simulink model "inv_rot_pen_RL_cntr_simscape_sim_1d_analysis"  (R2025b)
settings: Solver=FixedStepAuto  StartTime=0.0  StopTime=5  FixedStep=Ts  RelTol=1e-3
StopFcn:
  | myStopFcnAppendInitTime
values from neighbouring files (symbols this model uses):
  cfg = loaded.cfg    [continueFurutaMatlabSwingupTraining.m]    (also in evaluateFurutaController.m = makeFurutaConfig(); evaluateFurutaMatlabSwingupAgent.m = makeFurutaMatlabSwingupTD3Config(); finalizeFurutaDirectTD3Run.m = normalizeRunConfig(cfg, runDir); initFurutaSldrtHardwareWorkspace.m = makeFurutaMathWorksStyleWideTD3Config())
  i_max = 4    [initFurutaModelWorkspace.m]
  K = K_oben    [initFurutaModelWorkspace.m]
  Kp_i = db2mag(options.CurrentControllerKpDb)    [initFurutaModelWorkspace.m]    (also in initFurutaSldrtHardwareWorkspace.m = 2.5)
  omega0 = options.InitialOmega    [initFurutaModelWorkspace.m]
  param = get_parameter()    [initFurutaModelWorkspace.m]
  s = zpk("s")    [initFurutaModelWorkspace.m]    (also in initFurutaSldrtHardwareWorkspace.m)
  theta0 = options.InitialTheta    [initFurutaModelWorkspace.m]
  Tn_i = param.L / param.R    [initFurutaModelWorkspace.m]    (also in initFurutaSldrtHardwareWorkspace.m = 0.000286849073257)
  Ts_fast = cfg.Model.HardwareFastSampleTime    [initFurutaSldrtHardwareWorkspace.m]
undefined symbols (not defined in the file or in its folder): currentBias_A, currentNoiseStd_A, DiscIntNeverNeededParam, G_diff_theta1_ss, G_diff_theta2, G_diff_theta2_ss, G_encoder_notch_d_ss, rewardParams, safetyParams, X, Y, Z
libraries: sm_lib x57, nesl_utility x18, cstblocks x13, rllib x2, simulink x1
(part 3 of 3)

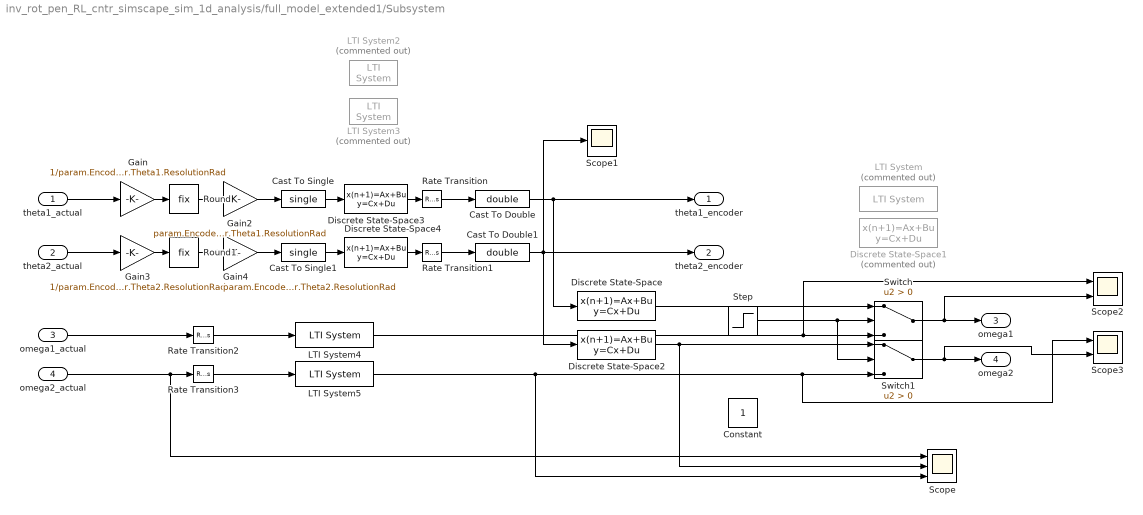
== system inv_rot_pen_RL_cntr_simscape_sim_1d_analysis/full_model_extended1/Subsystem ==
  theta1_actual : Inport
  theta2_actual : Inport  Port=2
  omega1_actual : Inport  Port=3
  omega2_actual : Inport  Port=4
  Cast To Double : DataTypeConversion  OutDataTypeStr=double  SaturateOnIntegerOverflow=off  RndMeth=Floor
  Cast To Double1 : DataTypeConversion  OutDataTypeStr=double  SaturateOnIntegerOverflow=off  RndMeth=Floor
  Cast To Single : DataTypeConversion  OutDataTypeStr=single  SaturateOnIntegerOverflow=off  RndMeth=Floor
  Cast To Single1 : DataTypeConversion  OutDataTypeStr=single  SaturateOnIntegerOverflow=off  RndMeth=Floor
  Constant : Constant
  Discrete State-Space : DiscreteStateSpace  A=G_diff_theta1_ss.A  B=G_diff_theta1_ss.B  C=G_diff_theta1_ss.C  D=G_diff_theta1_ss.D  InitialCondition=|  SampleTime=cfg.Agent.SampleTime
      | rampConsistentFilterX0( ...
      |     G_diff_theta1_ss, theta0(1), omega0(1), cfg.Agent.SampleTime);
  Discrete State-Space1 : DiscreteStateSpace  Commented=on  A=G_diff_theta2.A  B=G_diff_theta2.B  C=G_diff_theta2.C  D=G_diff_theta2.D  InitialCondition=2.78824  SampleTime=cfg.Agent.SampleTime
  Discrete State-Space2 : DiscreteStateSpace  A=G_diff_theta2_ss.A  B=G_diff_theta2_ss.B  C=G_diff_theta2_ss.C  D=G_diff_theta2_ss.D  InitialCondition=|  SampleTime=cfg.Agent.SampleTime
      | rampConsistentFilterX0( ...
      |     G_diff_theta2_ss, theta0(2), omega0(2), cfg.Agent.SampleTime);
  Discrete State-Space3 : DiscreteStateSpace  A=G_encoder_notch_d_ss.A  B=G_encoder_notch_d_ss.B  C=G_encoder_notch_d_ss.C  D=G_encoder_notch_d_ss.D  InitialCondition=|  SampleTime=Ts_fast
      | rampConsistentFilterX0( ...
      |     G_encoder_notch_d_ss, theta0(1), omega0(1), Ts_fast);
  Discrete State-Space4 : DiscreteStateSpace  A=G_encoder_notch_d_ss.A  B=G_encoder_notch_d_ss.B  C=G_encoder_notch_d_ss.C  D=G_encoder_notch_d_ss.D  InitialCondition=|  SampleTime=Ts_fast
      | rampConsistentFilterX0( ...
      |     G_encoder_notch_d_ss, theta0(2), omega0(2), Ts_fast);
  Gain : Gain  Gain=1/param.Encoder.Theta1.ResolutionRad
  Gain2 : Gain  Gain=param.Encoder.Theta1.ResolutionRad
  Gain3 : Gain  Gain=1/param.Encoder.Theta2.ResolutionRad
  Gain4 : Gain  Gain=param.Encoder.Theta2.ResolutionRad
  LTI System : cstblocks/LTI System  Commented=on  sys=G_diff_theta1  IC=[]  PadeOrder=0
  LTI System2 : cstblocks/LTI System  Commented=on  sys=G_encoder_notch_d  IC=[]  PadeOrder=0
  LTI System3 : cstblocks/LTI System  Commented=on  sys=G_encoder_notch_d  IC=[]  PadeOrder=0
  LTI System4 : cstblocks/LTI System  sys=G_filt_theta1  IC=[]  PadeOrder=0
  LTI System5 : cstblocks/LTI System  sys=G_filt_theta2  IC=[]  PadeOrder=0
  Rate Transition{,1..3} (4 alike) : RateTransition  OutPortSampleTime=cfg.Agent.SampleTime
  Round : Rounding  Operator=fix
  Round1 : Rounding  Operator=fix
  Scope : Scope  NumInputPorts=3
      settings: ActiveDisplayYMinimum=-19.570931470352093  ActiveDisplayYMaximum=24.355878033770182  DataLoggingVariableName=ScopeData11
  Scope1 : Scope
      settings: ActiveDisplayYMinimum=2.7442590296268463  ActiveDisplayYMaximum=3.1840349137783051  DataLoggingVariableName=ScopeData12
  Scope2 : Scope  NumInputPorts=2
      settings: ActiveDisplayYMinimum=-17.869651894957986  ActiveDisplayYMaximum=20.269813857281314  DataLoggingVariableName=ScopeData13
  Scope3 : Scope  NumInputPorts=2
      settings: ActiveDisplayYMinimum=-17.039216767214715  ActiveDisplayYMaximum=18.377458015393035  DataLoggingVariableName=ScopeData14
  Step : Step  Time=0  Before=-1  SampleTime=cfg.Agent.SampleTime
  Switch : Switch  Criteria=u2 > Threshold  SaturateOnIntegerOverflow=off  InputSameDT=off
  Switch1 : Switch  Criteria=u2 > Threshold  SaturateOnIntegerOverflow=off  InputSameDT=off
  theta1_encoder : Outport
  theta2_encoder : Outport  Port=2
  omega1 : Outport  Port=3
  omega2 : Outport  Port=4
  wires:
  Discrete State-Space4/1 -> Rate Transition1/1
  Discrete State-Space3/1 -> Rate Transition/1
  Cast To Single1/1 -> Discrete State-Space4/1
  Cast To Single/1 -> Discrete State-Space3/1
  Discrete State-Space/1 -> Switch/1
  theta2_actual/1 -> Gain3/1
  theta1_actual/1 -> Gain/1
  Gain3/1 -> Round1/1
  Gain4/1 -> Cast To Single1/1
  Gain/1 -> Round/1
  Round/1 -> Gain2/1
  Round1/1 -> Gain4/1
  Discrete State-Space2/1 -> Switch1/1, Scope/2
  Gain2/1 -> Cast To Single/1
  Cast To Double/1 -> Discrete State-Space/1, theta1_encoder/1
  Rate Transition/1 -> Cast To Double/1
  Rate Transition1/1 -> Cast To Double1/1
  Cast To Double1/1 -> Scope1/1, Discrete State-Space2/1, theta2_encoder/1
  omega1_actual/1 -> Rate Transition2/1
  Rate Transition2/1 -> LTI System4/1
  Switch1/1 -> Scope3/2, omega2/1
  Switch/1 -> Scope2/2, omega1/1
  Step/1 -> Switch1/2, Switch/2
  LTI System4/1 -> Scope2/1, Switch/3
  omega2_actual/1 -> Scope/1, Rate Transition3/1
  Rate Transition3/1 -> LTI System5/1
  LTI System5/1 -> Scope/3, Scope3/1, Switch1/3

== system inv_rot_pen_RL_cntr_simscape_sim_1d_analysis/full_model_extended1/Subsystem1 ==
  voltage_cmd : Inport
  Gain1 : Gain  Gain=2
  LTI System1 : cstblocks/LTI System  sys=G_pi_rolloff_d  IC=[]  PadeOrder=0
  Saturation : Saturate  UpperLimit=cfg.Limits.SupplyVoltage  LowerLimit=-cfg.Limits.SupplyVoltage
  Sign : Signum
  Sum1 : Sum  Inputs=++|
  voltage : Outport
  wires:
  LTI System1/1 -> Sum1/1, Sign/1
  Sign/1 -> Gain1/1
  voltage_cmd/1 -> LTI System1/1
  Sum1/1 -> Saturation/1
  Saturation/1 -> voltage/1

== system inv_rot_pen_RL_cntr_simscape_sim_1d_analysis/full_model_extended1/current noise ==
  current [A] : Inport
  Add : Sum  Inputs=+++
  Random Number : RandomNumber  SampleTime=cfg.Agent.SampleTime
  "currentBias_A " : Constant  Value=currentBias_A
  currentNoiseStd_A : Gain  Gain=currentNoiseStd_A
  current with noise [A] : Outport
  wires:
  current [A]/1 -> Add/1
  Add/1 -> current with noise [A]/1
  "currentBias_A "/1 -> Add/2
  Random Number/1 -> currentNoiseStd_A/1
  currentNoiseStd_A/1 -> Add/3

== matlab function inv_rot_pen_RL_cntr_simscape_sim_1d_analysis/Subsystem/Inverted Rotary Pendulum Analytical/MATLAB Function ==
  data: tau input size=1; alpha output size=[2,1]; theta input size=[2,1]; omega input size=[2,1]; param parameter
function alpha = fcn(tau, theta, omega, param)

    % M(q) * qdd + C(q,qdot) * qdot + G(q) + D * qdot = tau
    [M, C, G, D] = calculate_dynamics_furuta(theta, omega, param);
    alpha = M \ ( [tau; 0] - (C + D) * omega - G );

end

== matlab function inv_rot_pen_RL_cntr_simscape_sim_1d_analysis/rewardFunction/MATLAB Function ==
  data: obs input; u input; uPrev input; stepCount input; rewardParams parameter; r output; isDone output; safetyParams parameter; FurutaRewardDiagnosisBus output Bus: FurutaRewardDiagnosisBus; theta2_unwrapped input
function [r, isDone, FurutaRewardDiagnosisBus] = fcn(obs, u, uPrev, stepCount, rewardParams, safetyParams, theta2_unwrapped)
% params declared as block Parameter via Ports & Data Manager
[r, isDone, FurutaRewardDiagnosisBus] = rewardFcnFuruta(obs, u, uPrev, stepCount, rewardParams, safetyParams, theta2_unwrapped);
end

== matlab function inv_rot_pen_RL_cntr_simscape_sim_1d_analysis/full_model_extended/Inverted Rotary Pendulum Analytical with friction/MATLAB Function ==
  data: tau input size=1; alpha output size=[2,1]; theta input size=[2,1]; omega input size=[2,1]; param parameter
function alpha = fcn(tau, theta, omega, param)
% Physical Furuta plant dynamics with added joint friction.
%
% Input tau is the motor torque after current-loop / command compensation.
%
% M(q) qdd + C(q,qdot) qdot + G(q) + D qdot + tau_friction = tau_applied

    [M, C, G, D] = calculate_dynamics_furuta(theta, omega, param);

    tauFric1 = frictionTorque(omega(1), param.Friction.Theta1);

    % Start with theta1 friction only. Add theta2 later if evidence supports it.
    tauFric = [tauFric1; 0];

    alpha = M \ ([tau; 0] - (C + D) * omega - G - tauFric);

end

function tauF = frictionTorque(omega, fric)
% Smooth viscous + Coulomb/static friction model.
%
% tauF has the same sign as omega, so it opposes motion when subtracted from
% the applied generalized torque.

    viscous = fric.B * omega;

    coulombStatic = ...
        (fric.Tc + (fric.Ts - fric.Tc) * exp(-(abs(omega) / fric.OmegaS)^2)) * ...
        tanh(omega / fric.OmegaEps);

    %tauF = viscous + coulombStatic;
    %tauF = viscous*20 + coulombStatic;
    tauF = viscous*7 + coulombStatic*2.3; % looks to be the best overall
    %tauF = viscous*10 + coulombStatic*2.3;
end

== matlab function inv_rot_pen_RL_cntr_simscape_sim_1d_analysis/full_model_extended/Inverted Rotary Pendulum Analytical1/MATLAB Function ==
  data: tau input size=1; alpha output size=[2,1]; theta input size=[2,1]; omega input size=[2,1]; param parameter
function alpha = fcn(tau, theta, omega, param)

    % M(q) * qdd + C(q,qdot) * qdot + G(q) + D * qdot = tau
    [M, C, G, D] = calculate_dynamics_furuta(theta, omega, param);
    alpha = M \ ( [tau; 0] - (C + D) * omega - G );

end

== matlab function inv_rot_pen_RL_cntr_simscape_sim_1d_analysis/full_model_extended1/Inverted Rotary Pendulum Analytical with friction/MATLAB Function ==
  data: tau input size=1; alpha output size=[2,1]; theta input size=[2,1]; omega input size=[2,1]; param parameter
function alpha = fcn(tau, theta, omega, param)
% Physical Furuta plant dynamics with added joint friction.
%
% Input tau is the motor torque after current-loop / command compensation.
%
% M(q) qdd + C(q,qdot) qdot + G(q) + D qdot + tau_friction = tau_applied

    [M, C, G, D] = calculate_dynamics_furuta(theta, omega, param);

    tauFric1 = frictionTorque(omega(1), param.Friction.Theta1);

    % Start with theta1 friction only. Add theta2 later if evidence supports it.
    tauFric = [tauFric1; 0];

    alpha = M \ ([tau; 0] - (C + D) * omega - G - tauFric);

end

function tauF = frictionTorque(omega, fric)
% Smooth viscous + Coulomb/static friction model.
%
% tauF has the same sign as omega, so it opposes motion when subtracted from
% the applied generalized torque.

    viscous = fric.B * omega;

    coulombStatic = ...
        (fric.Tc + (fric.Ts - fric.Tc) * exp(-(abs(omega) / fric.OmegaS)^2)) * ...
        tanh(omega / fric.OmegaEps);

    %tauF = viscous + coulombStatic;
    %tauF = viscous*20 + coulombStatic;
    %tauF = viscous*7 + coulombStatic*2.3; % looks to be the best overall, when comparimg it vs 20260622_201704_hardware from results\model_vs_hardware\test1_constant_current_0p2a_disable_0p8s
    %tauF = viscous*7.5 + coulombStatic*2.3; % latest
    tauF = viscous*fric.viscousScalingFactor + coulombStatic*fric.coulombStaticScalingFactor;
end

== matlab function inv_rot_pen_RL_cntr_simscape_sim_1d_analysis/full_model_extended1/Inverted Rotary Pendulum Analytical1/MATLAB Function ==
  data: tau input size=1; alpha output size=[2,1]; theta input size=[2,1]; omega input size=[2,1]; param parameter
function alpha = fcn(tau, theta, omega, param)

    % M(q) * qdd + C(q,qdot) * qdot + G(q) + D * qdot = tau
    [M, C, G, D] = calculate_dynamics_furuta(theta, omega, param);
    alpha = M \ ( [tau; 0] - (C + D) * omega - G );

end
